simulink model "hw1_final"  (Simulink 7.9)
settings: Solver=ode45  StartTime=0.0  StopTime=10.0  RelTol=1e-3
settings Model: Creator=bazkoale  LastModifiedBy=alex
settings DataIOCC: SignalLoggingSaveFormat=Dataset
settings OptimizationCC: ExpressionDepthLimit=128
settings CodeAppCC: CustomSymbolStrType=$N$R$M_T

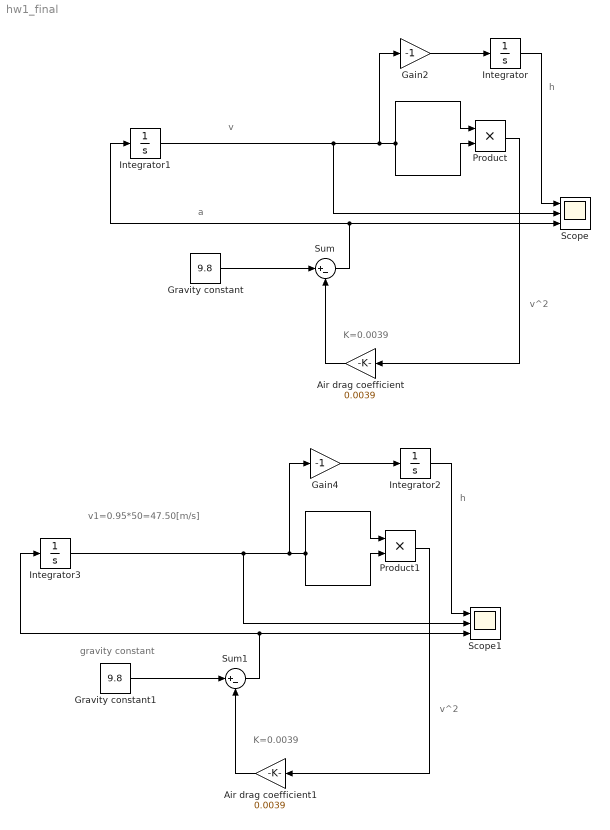
== system hw1_final ==
  note: v1=0.95*50=47.50[m/s]
  note: a
  note: v
  note: h
  note: h
  note: K=0.0039
  note: gravity constant
  note: v^2
  note: v^2
  note: K=0.0039
  Air drag coefficient : Gain  Gain=0.0039
  Air drag coefficient1 : Gain  Gain=0.0039
  Gain2 : Gain  Gain=-1
  Gain4 : Gain  Gain=-1
  Gravity constant : Constant  Value=9.8
  Gravity constant1 : Constant  Value=9.8
  Integrator : Integrator  InitialCondition=1000
  Integrator1 : Integrator  UpperSaturationLimit=47.5
  Integrator2 : Integrator  InitialCondition=1000
  Integrator3 : Integrator  LimitOutput=on  UpperSaturationLimit=47.5
  Product : Product
  Product1 : Product
  Scope : Scope  NumInputPorts=3
      settings: YMin=-5~-5~-5  YMax=5~5~5
  Scope1 : Scope  NumInputPorts=3
      settings: YMin=-5~-5~-5  YMax=5~5~5
  Sum : Sum  Inputs=|+-
  Sum1 : Sum  Inputs=|+-
  wires:
  Product/1 -> Air drag coefficient/1
  Sum/1 -> Integrator1/1, Scope/3
  Integrator/1 -> Scope/1
  Gravity constant/1 -> Sum/1
  Air drag coefficient/1 -> Sum/2
  Integrator1/1 -> Scope/2, Gain2/1, Product/1, Product/2
  Gain2/1 -> Integrator/1
  Product1/1 -> Air drag coefficient1/1
  Sum1/1 -> Integrator3/1, Scope1/3
  Integrator2/1 -> Scope1/1
  Gravity constant1/1 -> Sum1/1
  Air drag coefficient1/1 -> Sum1/2
  Integrator3/1 -> Scope1/2, Gain4/1, Product1/1, Product1/2
  Gain4/1 -> Integrator2/1
